simulink model "jetVane6DOFSimulation"  (R2022b)
settings: Solver=VariableStepAuto  StartTime=0.0  StopTime=SIM_TIME  RelTol=1e-3
values from neighbouring files (symbols this model uses):
  x0 = [0 ... (first row only)    [initialize.m]
undefined symbols (not defined in the file or in its folder): rocket_model
settings Model: Creator=alber  LastModifiedBy=alber

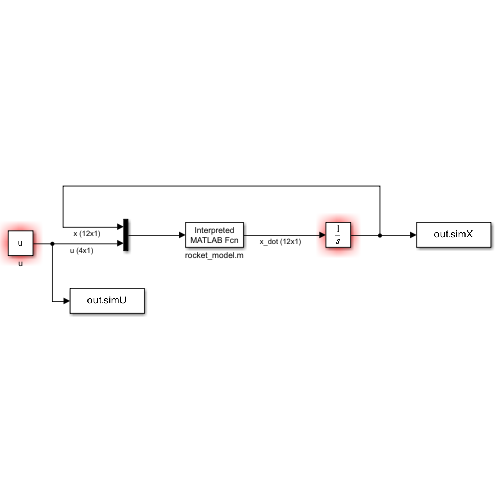
[thumbnail: Simulink's stored preview of the top-level diagram]
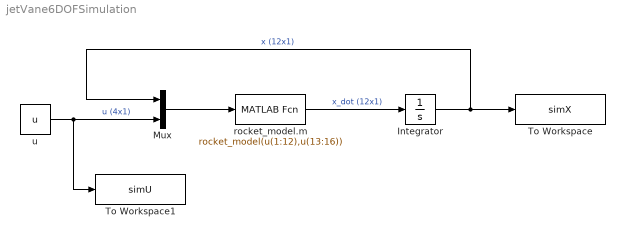
== system jetVane6DOFSimulation ==
  Integrator : Integrator  InitialCondition=x0
  Mux : Mux  Inputs=2
  To Workspace : ToWorkspace  VariableName=simX  SaveFormat=Timeseries  SampleTime=-1
  To Workspace1 : ToWorkspace  VariableName=simU  SaveFormat=Timeseries  SampleTime=-1
  rocket_model.m : MATLABFcn  MATLABFcn=rocket_model(u(1:12),u(13:16))
  u : Constant  Value=u
  wires:
  Integrator/1 -> Mux/1, To Workspace/1  "x (12x1)"
  rocket_model.m/1 -> Integrator/1  "x_dot (12x1)"
  u/1 -> To Workspace1/1, Mux/2  "u (4x1)"
  Mux/1 -> rocket_model.m/1
